simulink model "New_SinglePulseModel_n_B8"  (R2014b)
settings: Solver=FixedStepDiscrete  StartTime=0.0  StopTime=200  RelTol=1e-3
InitFcn:
  | initialization_new;
values from neighbouring files (symbols this model uses):
  PCtimings1 = [0:1:30]*1e-9    [initialization_new.m]    (also in initialization_pulsePicking.m = PCtimings1; runModel.m = [PCtimings1 onTime offTime]; runPulsePickingModel.m = [PCtimings1 onTime offTime]; simulate_over_NT.m = [])
  PCtimings2 = [0]*1e-9    [initialization_new.m]    (also in simulate_over_NT.m = [])
libraries: BlockLib x20, dspsrcs4 x1
settings Model: Creator=Alexander  LastModifiedBy=kunalmenda

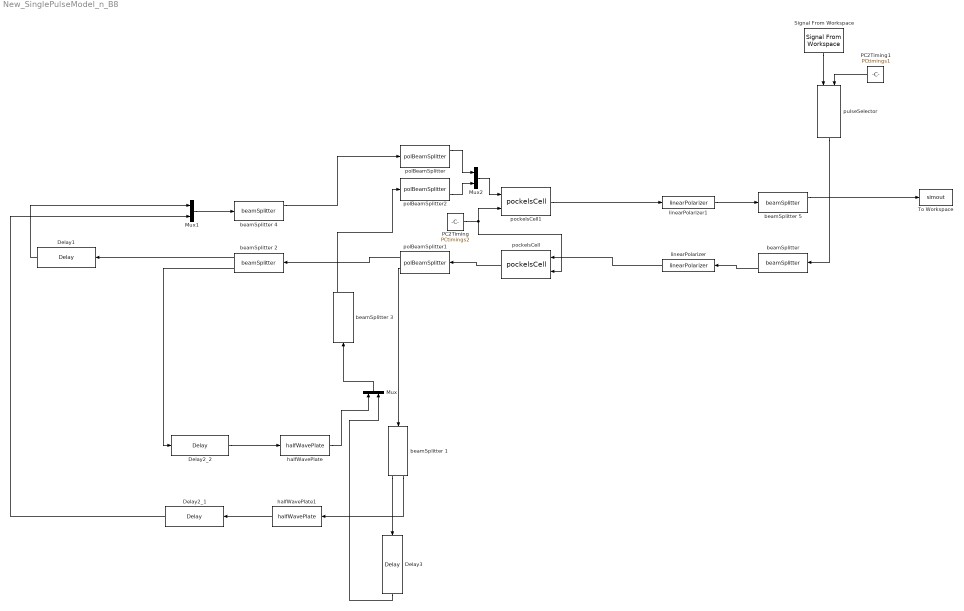
== system New_SinglePulseModel_n_B8 ==
  Delay1 : BlockLib/Delay  DelayAmt=10e-9
  Delay2_1 : BlockLib/Delay  DelayAmt=14.33e-9
  Delay2_2 : BlockLib/Delay  DelayAmt=14.33e-9
  Delay3 : BlockLib/Delay  DelayAmt=18.66e-9
  Mux : Mux  Inputs=2
  Mux1 : Mux  Inputs=2
  Mux2 : Mux  Inputs=2
  PC2Timing : Constant  Value=PCtimings2
  PC2Timing1 : Constant  Value=PCtimings1
  Signal From Workspace : dspsrcs4/Signal From Workspace  X=inputsignal  Ts=1  nsamps=1  OutputAfterFinalValue=Setting to zero  ignoreOrWarnInputAndFrameLengths=off
  To Workspace : ToWorkspace  VariableName=simout  SaveFormat=Timeseries  SampleTime=-1
  beamSplitter {,1..5} (6 alike) : BlockLib/beamSplitter 
  halfWavePlate : BlockLib/halfWavePlate  AxisAngle=pi/4
  halfWavePlate1 : BlockLib/halfWavePlate  AxisAngle=pi/4
  linearPolarizer : BlockLib/linearPolarizer  AxisAngle=pi/2
  linearPolarizer1 : BlockLib/linearPolarizer  AxisAngle=pi/2
  pockelsCell : BlockLib/pockelsCell  OutputDimensions=1  AxisAngle=pi/4
  pockelsCell1 : BlockLib/pockelsCell  OutputDimensions=4  AxisAngle=pi/4
  polBeamSplitter : BlockLib/polBeamSplitter
  polBeamSplitter1 : BlockLib/polBeamSplitter
  polBeamSplitter2 : BlockLib/polBeamSplitter
  pulseSelector : BlockLib/pulseSelector  OutputDimensions=1
  wires:
  pulseSelector/1 -> "beamSplitter "/1
  polBeamSplitter1/2 -> beamSplitter 1/1
  polBeamSplitter1/1 -> beamSplitter 2/1
  beamSplitter 2/1 -> Delay1/1
  beamSplitter 1/1 -> Delay3/1
  beamSplitter 1/2 -> halfWavePlate1/1
  halfWavePlate1/1 -> Delay2_1/1
  Delay2_1/1 -> Mux1/2
  Delay3/1 -> Mux/2
  Mux/1 -> beamSplitter 3/1
  halfWavePlate/1 -> Mux/1
  Mux1/1 -> beamSplitter 4/1
  Delay1/1 -> Mux1/1
  beamSplitter 4/1 -> polBeamSplitter/1
  beamSplitter 3/1 -> polBeamSplitter2/1
  Signal From Workspace/1 -> pulseSelector/1
  Delay2_2/1 -> halfWavePlate/1
  pockelsCell1/1 -> linearPolarizer1/1
  linearPolarizer1/1 -> beamSplitter 5/1
  PC2Timing/1 -> pockelsCell1/2, pockelsCell/2
  "beamSplitter "/2 -> linearPolarizer/1
  beamSplitter 2/2 -> Delay2_2/1
  PC2Timing1/1 -> pulseSelector/2
  linearPolarizer/1 -> pockelsCell/1
  pockelsCell/1 -> polBeamSplitter1/1
  beamSplitter 5/1 -> To Workspace/1
  polBeamSplitter/1 -> Mux2/1
  polBeamSplitter2/2 -> Mux2/2
  Mux2/1 -> pockelsCell1/1
